simulink model "ric_serie"  (R2015a)
settings: Solver=ode45  StartTime=0.0  StopTime=10.0  RelTol=1e-6  AbsTol=1e-6
values from neighbouring files (symbols this model uses):
  C = 8.0e-1    (= 0.8)    [var_elser.m]
undefined symbols (not defined in the file or in its folder): L, R, V
libraries: fl_lib x6, nesl_utility x3
settings Model: Creator=11802972  LastModifiedBy=11802972

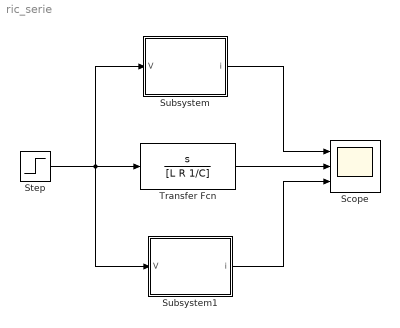
== system ric_serie ==
  Scope : Scope  NumInputPorts=3
      settings: YMin=-5~-5~-5  YMax=5~5~5
  Step : Step  After=V  SampleTime=0
  Subsystem : Subsystem
  Subsystem1 : Subsystem
  Transfer Fcn : TransferFcn  Numerator=[1 0]  Denominator=[L R 1/C]
  wires:
  Step/1 -> Subsystem1/1(V), Subsystem/1(V), Transfer Fcn/1
  Subsystem/1(i) -> Scope/1
  Transfer Fcn/1 -> Scope/2
  Subsystem1/1(i) -> Scope/3

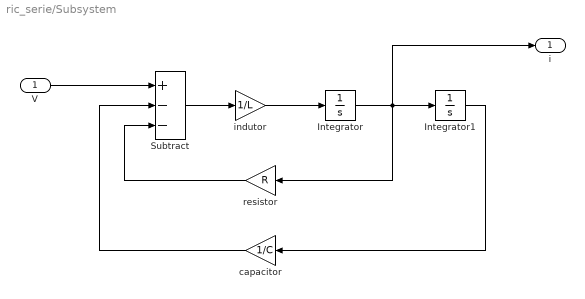
== system ric_serie/Subsystem ==
  V : Inport
  Integrator : Integrator
  Integrator1 : Integrator
  Subtract : Sum  Inputs=+--
  capacitor : Gain  Gain=1/C
  indutor : Gain  Gain=1/L
  resistor : Gain  Gain=R
  i : Outport
  wires:
  Subtract/1 -> indutor/1
  V/1 -> Subtract/1
  resistor/1 -> Subtract/3
  Integrator/1 -> i/1, resistor/1, Integrator1/1
  capacitor/1 -> Subtract/2
  Integrator1/1 -> capacitor/1
  indutor/1 -> Integrator/1

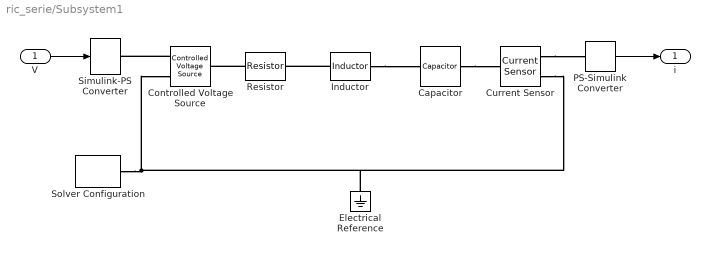
== system ric_serie/Subsystem1 ==
  V : Inport
  Capacitor : fl_lib/Electrical/Electrical Elements/Capacitor  c=C F  r=0 Ohm  g=0 1/Ohm  i_specify=off  i_priority=High  i=0 A  v_specify=off  v_priority=High  v=0 V  vc_specify=off  vc_priority=High  vc=0 V
  Controlled Voltage Source : fl_lib/Electrical/Electrical Sources/Controlled Voltage Source
  Current Sensor : fl_lib/Electrical/Electrical Sensors/Current Sensor
  Electrical Reference : fl_lib/Electrical/Electrical Elements/Electrical Reference
  Inductor : fl_lib/Electrical/Electrical Elements/Inductor  l=L H  r=0 Ohm  g=0 1/Ohm  i_specify=off  i_priority=High  i=0 A  v_specify=off  v_priority=High  v=0 V  i_L_specify=off  i_L_priority=High  i_L=0 A
  PS-Simulink Converter : nesl_utility/PS-Simulink Converter  PhysicalDomain=network_engine_domain  SubClassName=ps_output  LeftPortType=input  RightPortType=output  PseudoPeriodic=off  Frequencies=[]  Unit=1  AffineConversion=off
  Resistor : fl_lib/Electrical/Electrical Elements/Resistor  R=R Ohm  i_specify=off  i_priority=High  i=0 A  v_specify=off  v_priority=High  v=0 V
  Simulink-PS Converter : nesl_utility/Simulink-PS Converter  PhysicalDomain=network_engine_domain  SubClassName=ps_input  LeftPortType=input  RightPortType=output  PseudoPeriodic=off  Frequencies=[]  NoiseDistribution=none  NoiseParameters=[]  Unit=1  AffineConversion=off  InputFiltering=off  SimscapeFilterOrder=1  InputFilterTimeConstant=0.001  UdotUserProvided=1
  Solver Configuration : nesl_utility/Solver Configuration  PhysicalDomain=network_engine_domain  SubClassName=solver  LeftPortType=input  RightPortType=generic  Accelerate=off  Tones=[]  Harmonics=[]  SimulateNoise=off  Profile=off  UseLocalSampling=off  EnableSwitchedLinearOptims=on  FrequencyDomain=off  UseCCode=off  RelTol=0.001  AbsTol=1e-06  MinStep=1e-09  ToWorkspace=off  RevertToSquareIcSolve=off  NumHomotopyIterations=100  DoDC=off  ResidualTolerance=1e-06  UseLocalSolver=off  LocalSolverChoice=NE_BACKWARD_EULER_ADVANCER  LocalSolverSampleTime=0.001  DoFixedCost=off  MaxNonlinIter=3  MaxModeIter=2  LinearAlgebra=Sparse  DelaysMemoryBudget=1024  AutomaticFiltering=on  FilteringTimeConstant=0.001
  i : Outport
  wires:
  PS-Simulink Converter/1 -> i/1
  V/1 -> Simulink-PS Converter/1
  connections:
  Controlled Voltage Source/RConn1 -- Simulink-PS Converter/RConn1
  Current Sensor/RConn1 -- PS-Simulink Converter/LConn1
  Resistor/LConn1 -- Controlled Voltage Source/LConn1
  Capacitor/RConn1 -- Current Sensor/LConn1
  Inductor/RConn1 -- Capacitor/LConn1
  Inductor/LConn1 -- Resistor/RConn1
  Solver Configuration/RConn1 -- Current Sensor/RConn2 -- Electrical Reference/LConn1 -- Controlled Voltage Source/RConn2
